simulink model "DynamicsModel"  (R2019a)
settings: Solver=VariableStepAuto  StartTime=0.0  StopTime=600  MaxStep=10.0  RelTol=1e-3
libraries: simulink x4, aerolibatmos2 x1
settings Model: Creator=Daniel  LastModifiedBy=Daniel
settings DataIOCC: ReturnWorkspaceOutputs=off
settings DebuggingCC: PregeneratedLibrarySubsystemCodeDiagnostic=none  ArithmeticOperatorsInVariantConditions=warning
settings SFSimCC: SimUseLocalCustomCode=off
settings RTWCC: RTWUseLocalCustomCode=off

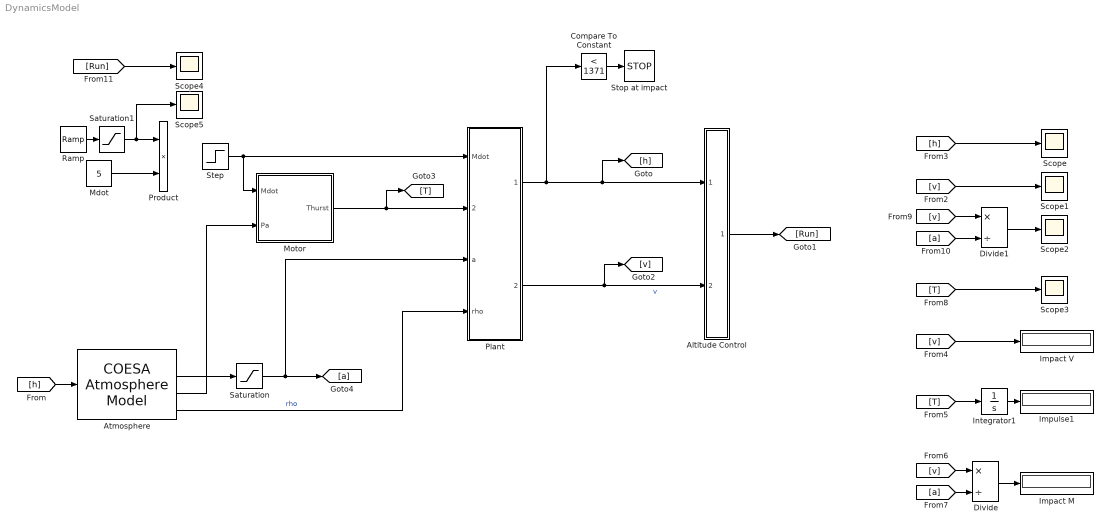
== system DynamicsModel ==
  Altitude Control : Subsystem
  "Atmosphere " : aerolibatmos2/COESA Atmosphere Model  units=Metric (MKS)  spec=1976 COESA-extended U.S. Standard Atmosphere  model=Profile  profile_var=High temperature  profile_percent=1%  profile_alt=5 km (16404 ft)  envelope_var=High temperature  envelope_percent=1%  action=Warning
  Compare To Constant : simulink/Logic and Bit Operations/Compare To Constant  relop=<  const=1371  OutDataTypeStr=boolean
  Divide : Product  Inputs=*/
  Divide1 : Product  Inputs=*/
  Impact M : Display
  Impact V : Display
  Impulse1 : Display
  Integrator1 : Integrator
  Mdot : Constant  Value=5
  Motor : Subsystem
  Plant : Subsystem
  Product : Product
  Ramp : simulink/Sources/Ramp  slope=-1000  start=72  InitialOutput=1
  Saturation : Saturate  UpperLimit=inf  LowerLimit=1
  Saturation1 : Saturate  UpperLimit=inf  LowerLimit=0
  Scope{,1..5} (6 alike) : Scope
  Step : Step  Time=70  Before=5  After=0  SampleTime=0
  Stop at impact : Stop
  wires:
  Plant/1(Altitude) -> Altitude Control/1(h), [h], Compare To Constant/1
  [h] -> "Atmosphere "/1
  "Atmosphere "/4 -> Plant/4(rho)  "rho"
  Plant/2("Velocity ") -> Altitude Control/2(v), [v]  "v"
  Compare To Constant/1 -> Stop at impact/1
  [v] -> Scope1/1
  [h] -> Scope/1
  [v] -> Impact V/1
  Integrator1/1 -> Impulse1/1
  [T] -> Integrator1/1
  [v] -> Divide/1
  Divide/1 -> Impact M/1
  "Atmosphere "/2 -> Saturation/1
  [a] -> Divide/2
  Divide1/1 -> Scope2/1
  [v] -> Divide1/1
  Altitude Control/1(Run) -> [Run]
  "Atmosphere "/3 -> Motor/2(Pa)
  [T] -> Scope3/1
  Mdot/1 -> Product/2
  [a] -> Divide1/2
  Saturation/1 -> [a], Plant/3(a)
  [Run] -> Scope4/1
  Motor/1(Thurst) -> [T], Plant/2("Thrust ")
  Ramp/1 -> Saturation1/1
  Saturation1/1 -> Scope5/1, Product/1
  Step/1 -> Plant/1(Mdot), Motor/1(Mdot)

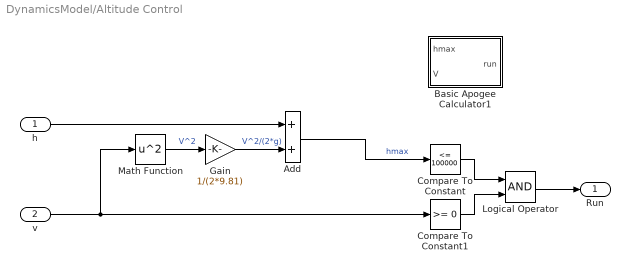
== system DynamicsModel/Altitude Control ==
  h : Inport
  v : Inport  Port=2
  Add : Sum
  Basic Apogee Calculator1 : MATLAB Function  TreatAsAtomicUnit=on
  Compare To Constant : simulink/Logic and Bit Operations/Compare To Constant  relop=<=  const=100000  OutDataTypeStr=boolean
  Compare To Constant1 : simulink/Logic and Bit Operations/Compare To Constant  relop=>=  const=0  OutDataTypeStr=boolean
  Gain : Gain  Gain=1/(2*9.81)
  Logical Operator : Logic  AllPortsSameDT=off  OutDataTypeStr=boolean
  Math Function : Math  Operator=square  SaturateOnIntegerOverflow=on
  Run : Outport
  wires:
  Math Function/1 -> Gain/1  "V^2"
  Add/1 -> Compare To Constant/1  "hmax"
  h/1 -> Add/1
  Gain/1 -> Add/2  "V^2/(2*g)"
  v/1 -> Compare To Constant1/1, Math Function/1
  Logical Operator/1 -> Run/1
  Compare To Constant/1 -> Logical Operator/1
  Compare To Constant1/1 -> Logical Operator/2

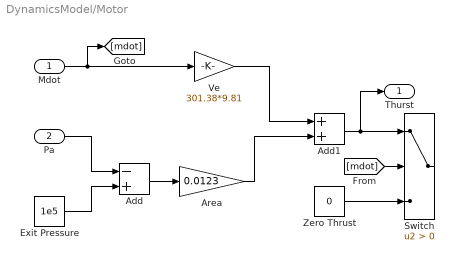
== system DynamicsModel/Motor ==
  Mdot : Inport
  Pa : Inport  Port=2
  Add : Sum  Inputs=-+
  Add1 : Sum
  Area : Gain  Gain=0.0123
  Exit Pressure : Constant  Value=1e5
  Switch : Switch  Criteria=u2 > Threshold
  "Ve " : Gain  Gain=301.38*9.81
  Zero Thrust : Constant  Value=0
  Thurst : Outport
  wires:
  Exit Pressure/1 -> Add/2
  Add/1 -> Area/1
  "Ve "/1 -> Add1/1
  Pa/1 -> Add/1
  Add1/1 -> Thurst/1, Switch/1
  Zero Thrust/1 -> Switch/3
  [mdot] -> Switch/2
  Area/1 -> Add1/2
  Mdot/1 -> [mdot], "Ve "/1

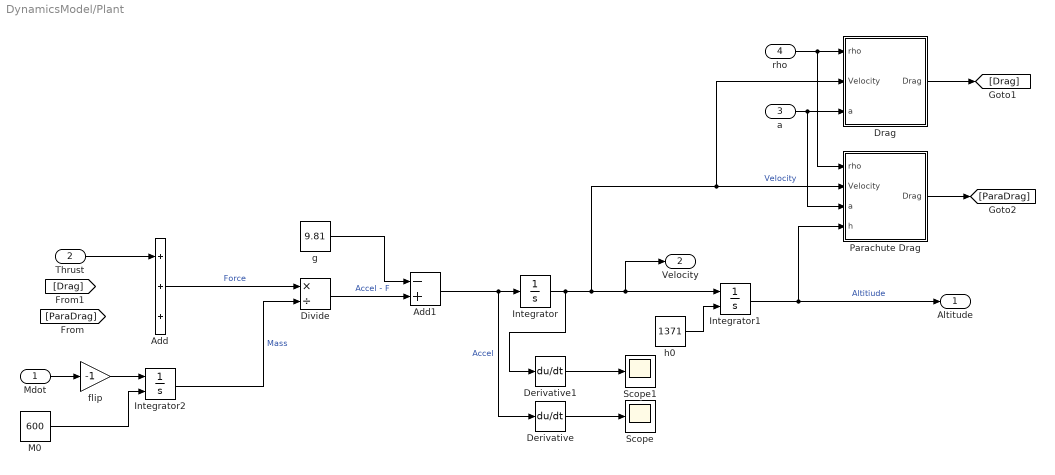
== system DynamicsModel/Plant ==
  Mdot : Inport
  "Thrust " : Inport  Port=2
  a : Inport  Port=3
  rho : Inport  Port=4
  Add : Sum  Inputs=+++
  Add1 : Sum  Inputs=-+
  Derivative : Derivative
  Derivative1 : Derivative
  Divide : Product  Inputs=*/
  Drag : Subsystem
  Integrator : Integrator  UpperSaturationLimit=5000  LowerSaturationLimit=-5000  ContinuousStateAttributes='Velocity'
  Integrator1 : Integrator  InitialConditionSource=external  LowerSaturationLimit=0
  Integrator2 : Integrator  InitialConditionSource=external
  M0 : Constant  Value=600
  Parachute Drag : Subsystem
  Scope : Scope
  Scope1 : Scope
  "flip " : Gain  Gain=-1
  g : Constant  Value=9.81
  h0 : Constant  Value=1371
  Altitude : Outport
  "Velocity " : Outport  Port=2
  wires:
  Integrator1/1 -> Parachute Drag/4(h), Altitude/1  "Altitiude"
  M0/1 -> Integrator2/2
  Add/1 -> Divide/1  "Force"
  Integrator2/1 -> Divide/2  "Mass"
  Integrator/1 -> Derivative1/1, Drag/2(Velocity), Parachute Drag/2(Velocity), "Velocity "/1, Integrator1/1  "Velocity"
  Add1/1 -> Derivative/1, Integrator/1  "Accel"
  Divide/1 -> Add1/2  "Accel - F"
  g/1 -> Add1/1
  Drag/1(Drag) -> [Drag]
  Mdot/1 -> "flip "/1
  "Thrust "/1 -> Add/1
  rho/1 -> Parachute Drag/1("rho "), Drag/1("rho ")
  "flip "/1 -> Integrator2/1
  a/1 -> Parachute Drag/3(a), Drag/3(a)
  h0/1 -> Integrator1/2
  Parachute Drag/1(Drag) -> [ParaDrag]
  Derivative/1 -> Scope/1
  Derivative1/1 -> Scope1/1

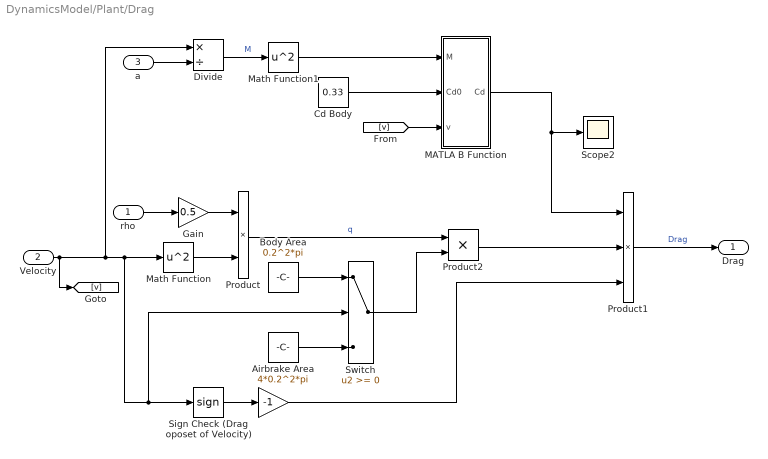
== system DynamicsModel/Plant/Drag ==
  "rho " : Inport
  Velocity : Inport  Port=2
  a : Inport  Port=3
  " " : Gain  Gain=-1
  Airbrake Area : Constant  Value=4*0.2^2*pi
  Body Area : Constant  Value=0.2^2*pi
  Cd Body : Constant  Value=0.33
  Divide : Product  Inputs=*/
  Gain : Gain  Gain=0.5
  MATLA B Function : MATLAB Function  TreatAsAtomicUnit=on
  Math Function : Math  Operator=square  SaturateOnIntegerOverflow=on
  Math Function1 : Math  Operator=square  SaturateOnIntegerOverflow=on
  Product : Product
  Product1 : Product  Inputs=3
  Product2 : Product
  Scope2 : Scope
  "Sign Check (Drag oposet of Velocity) " : Signum
  Switch : Switch
  Drag : Outport
  wires:
  Product1/1 -> Drag/1  "Drag"
  Gain/1 -> Product/1
  Math Function/1 -> Product/2
  "rho "/1 -> Gain/1
  "Sign Check (Drag oposet of Velocity) "/1 -> " "/1
  Velocity/1 -> [v], Divide/1, Switch/2, "Sign Check (Drag oposet of Velocity) "/1, Math Function/1
  a/1 -> Divide/2
  Divide/1 -> Math Function1/1  "M"
  Math Function1/1 -> MATLA B Function/1(M)
  Cd Body/1 -> MATLA B Function/2(Cd0)
  MATLA B Function/1(Cd) -> Scope2/1, Product1/1
  " "/1 -> Product1/3
  Product2/1 -> Product1/2
  Product/1 -> Product2/1  "q"
  Switch/1 -> Product2/2
  Body Area/1 -> Switch/1
  Airbrake Area/1 -> Switch/3
  [v] -> MATLA B Function/3(v)

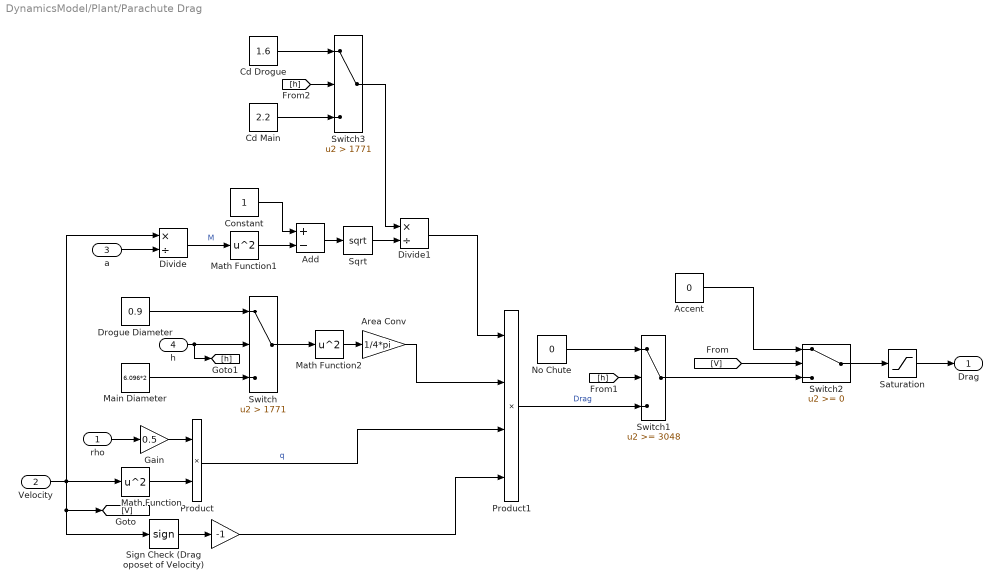
== system DynamicsModel/Plant/Parachute Drag ==
  "rho " : Inport
  Velocity : Inport  Port=2
  a : Inport  Port=3
  h : Inport  Port=4
  " " : Gain  Gain=-1
  Accent : Constant  Value=0
  Add : Sum  Inputs=+-
  Area Conv : Gain  Gain=1/4*pi
  Cd Drogue : Constant  Value=1.6
  Cd Main : Constant  Value=2.2
  Constant : Constant
  Divide : Product  Inputs=*/
  Divide1 : Product  Inputs=*/
  Drogue Diameter : Constant  Value=0.9
  Gain : Gain  Gain=0.5
  "Main Diameter " : Constant  Value=6.096*2
  Math Function : Math  Operator=square  SaturateOnIntegerOverflow=on
  Math Function1 : Math  Operator=square  SaturateOnIntegerOverflow=on
  Math Function2 : Math  Operator=square  SaturateOnIntegerOverflow=on
  No Chute : Constant  Value=0
  Product : Product
  Product1 : Product  Inputs=4
  Saturation : Saturate  UpperLimit=5e4  LowerLimit=-5e4
  "Sign Check (Drag oposet of Velocity) " : Signum
  Sqrt : Sqrt  SaturateOnIntegerOverflow=on
  Switch : Switch  Criteria=u2 > Threshold  Threshold=1771
  Switch1 : Switch  Threshold=3048
  Switch2 : Switch
  Switch3 : Switch  Criteria=u2 > Threshold  Threshold=1771
  Drag : Outport
  wires:
  Divide1/1 -> Product1/1
  Math Function1/1 -> Add/2
  Divide/1 -> Math Function1/1  "M"
  a/1 -> Divide/2
  Velocity/1 -> Math Function/1, "Sign Check (Drag oposet of Velocity) "/1, [V], Divide/1
  "Sign Check (Drag oposet of Velocity) "/1 -> " "/1
  "rho "/1 -> Gain/1
  Math Function/1 -> Product/2
  Gain/1 -> Product/1
  Constant/1 -> Add/1
  Add/1 -> Sqrt/1
  " "/1 -> Product1/4
  Product/1 -> Product1/3  "q"
  Drogue Diameter/1 -> Switch/1
  "Main Diameter "/1 -> Switch/3
  h/1 -> Switch/2, [h]
  Switch/1 -> Math Function2/1
  Math Function2/1 -> Area Conv/1
  Area Conv/1 -> Product1/2
  No Chute/1 -> Switch1/1
  Product1/1 -> Switch1/3  "Drag"
  Accent/1 -> Switch2/1
  Switch1/1 -> Switch2/3
  [V] -> Switch2/2
  Switch2/1 -> Saturation/1
  [h] -> Switch1/2
  Sqrt/1 -> Divide1/2
  Saturation/1 -> Drag/1
  Cd Main/1 -> Switch3/3
  Cd Drogue/1 -> Switch3/1
  [h] -> Switch3/2
  Switch3/1 -> Divide1/1

== matlab function DynamicsModel/Plant/Drag/MATLA B Function ==
  data: M input; Cd output; Cd0 input; v input
function Cd = fcn(M, Cd0, v)

    if (abs(M) < 1)
        Cd = Cd0/sqrt(1 - M);
    else
        Cd = Cd0/sqrt(M - 1);
    end
    
    if (v < 0)
        Cd = 1.28
    end

== matlab function DynamicsModel/Altitude Control/Basic Apogee Calculator1 ==
  data: hmax input; V input; run output
function run = fcn(hmax, V)

%Shut down motor when predicted apogee is over 100 km
if(hmax <= 100000 && V >= 0)
    run = 1;
else
    run = 0;
end
